simulink model "TestHarness_RotateTransform"  (R2020b)
settings: Solver=FixedStepAuto  StartTime=0.0  StopTime=0.1  FixedStep=0.1  RelTol=1e-3
settings Model: Creator=tomonori  LastModifiedBy=tomonori
settings DataIOCC: SaveOutput=off  SignalLogging=off  DSMLogging=off  SaveTime=off  ReturnWorkspaceOutputs=off

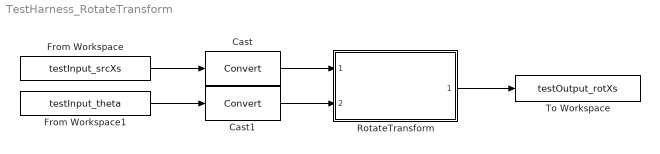
== system TestHarness_RotateTransform ==
  Cast : DataTypeConversion
  Cast1 : DataTypeConversion
  From Workspace : FromWorkspace  VariableName=testInput_srcXs
  From Workspace1 : FromWorkspace  VariableName=testInput_theta
  RotateTransform : Subsystem  ReferencedSubsystem=RotateTransform
  To Workspace : ToWorkspace  VariableName=testOutput_rotXs  SaveFormat=Timeseries  SampleTime=-1
  wires:
  From Workspace/1 -> Cast/1
  From Workspace1/1 -> Cast1/1
  Cast/1 -> RotateTransform/1
  Cast1/1 -> RotateTransform/2
  RotateTransform/1 -> To Workspace/1
